simulink model "command_handler"  (Simulink 8.2)
settings: Solver=ode1  StartTime=0.0  StopTime=Inf  FixedStep=0.001  RelTol=1e-3
PostLoadFcn:
  | , if any(exist('dsrtsu_mdlpostloadfcn', 'file') == [2, 3, 6]), try dsrtsu_mdlpostloadfcn('Execute', bdroot); catch fprintf('Error in PostLoadFcn (dsrtsu_mdlpostloadfcn) for model "%s":\n %s\n', bdroot, lasterr); end, end,
settings Model: DSRTSU_INTERNAL_RTI_VER=450  DSRTSU_INTERNAL_RTI_TYPE=rti1401  Creator=rushk1  LastModifiedBy=rushk1  BufferReuse=off
settings DataIOCC: SignalLoggingSaveFormat=Dataset
settings OptimizationCC: BlockReduction=off  OptimizeBlockIOStorage=off  BufferReuse=off  ExpressionFolding=off  ExpressionDepthLimit=128  LocalBlockOutputs=off
settings DebuggingCC: FcnCallInpInsideContextMsg=EnableAllAsError  StateNameClashWarn=none
settings RTWCC: SystemTargetFile=rti1401.tlc  MakeCommand=make_rti  TemplateMakefile=rti1401.tmf  Description=dSPACE DS1401 Hardware Platform  ProcessScript=rti1401_make_rtw_hook
settings STFCustomTargetCC: CodeReplacementLibrary=ANSI_C  ModelReferenceCompliant=off  ParMdlRefBuildCompliant=on  GeneratePreprocessorConditionals=Disable all  MatFileLogging=on  SystemTargetFile=rti1401.tlc
settings GRTTargetCC: ModelReferenceCompliant=off  CompOptLevelCompliant=off  ConcurrentExecutionCompliant=off
settings CustomProperty: DataType=RTWOptions_EnumType_C__Program Files_dSPACE RCPHIL 2014-B_MATLAB_RTI_RTI1401_TLC_rti1401_1InitialSimState  Value=RUN
settings EnumStrPairs: String=RUN

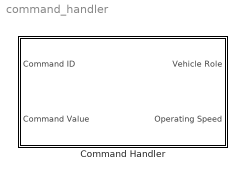
== system command_handler ==
  Command Handler : Subsystem

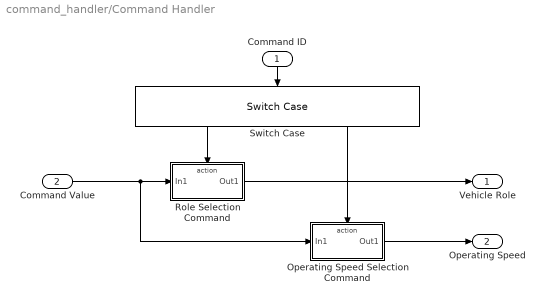
== system command_handler/Command Handler ==
  Command ID : Inport
  Command Value : Inport  Port=2
  Operating Speed Selection Command : Subsystem  TreatAsAtomicUnit=on
  Role Selection Command : Subsystem  TreatAsAtomicUnit=on
  Switch Case : SwitchCase  CaseConditions={129, 130}  ShowDefaultCase=off
  Vehicle Role : Outport
  Operating Speed : Outport  Port=2
  wires:
  Command ID/1 -> Switch Case/1
  Switch Case/1 -> Role Selection Command/Action
  Switch Case/2 -> Operating Speed Selection Command/Action
  Command Value/1 -> Operating Speed Selection Command/1(In1), Role Selection Command/1(In1)
  Operating Speed Selection Command/1(Out1) -> Operating Speed/1
  Role Selection Command/1(Out1) -> Vehicle Role/1

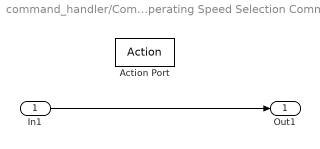
== system command_handler/Command Handler/Operating Speed Selection Command ==
  In1 : Inport
  Action Port : ActionPort  ActionType=case
  Out1 : Outport
  wires:
  In1/1 -> Out1/1

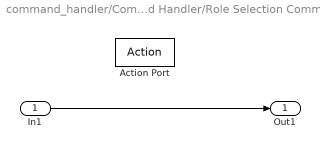
== system command_handler/Command Handler/Role Selection Command ==
  In1 : Inport
  Action Port : ActionPort  ActionType=case
  Out1 : Outport
  wires:
  In1/1 -> Out1/1
